simulink model "Total_90_NCKH"  (R2016a)
settings: Solver=FixedStepAuto  StartTime=0.0  StopTime=inf  RelTol=1e-3
libraries: arduinolib x12
settings Model: SimulationMode=external  ExtModeTrigDuration=2  Creator=Khuu Bach Thy  LastModifiedBy=ACER
settings OptimizationCC: OptimizeModelRefInitCode=on  LifeSpan=Inf  MaxStackSize=64
settings HardwareCC: ProdBitPerPointer=32  ProdLargestAtomicInteger=Long  ProdLargestAtomicFloat=Double  ProdWordSize=32  ProdHWDeviceType=ARM Compatible->ARM Cortex
settings RTWCC: SystemTargetFile=ert.tlc  HardwareBoard=Arduino Due  TemplateMakefile=ert_default_tmf  GenerateReport=on  Toolchain=Arduino ARM v1.6.1  BuildConfiguration=Faster Runs  IncludeHyperlinkInReport=on  LaunchReport=on  GenerateTraceInfo=on  GenerateTraceReport=on  GenerateTraceReportSl=on  GenerateTraceReportSf=on  GenerateTraceReportEml=on
settings CodeAppCC: ForceParamTrailComments=on  IgnoreCustomStorageClasses=off  OperatorAnnotations=on  SimulinkDataObjDesc=on  SFDataObjDesc=on  MATLABFcnDesc=on  MangleLength=10  InsertBlockDesc=on  MATLABSourceComments=on
settings ERTTargetCC: SupportContinuousTime=on  SupportVariableSizeSignals=on  ExtMode=on  ExtModeTransport=3  ExtModeMexFile=ext_serial_win32_comm_rtt  ExtModeMexArgs=0 10 115200

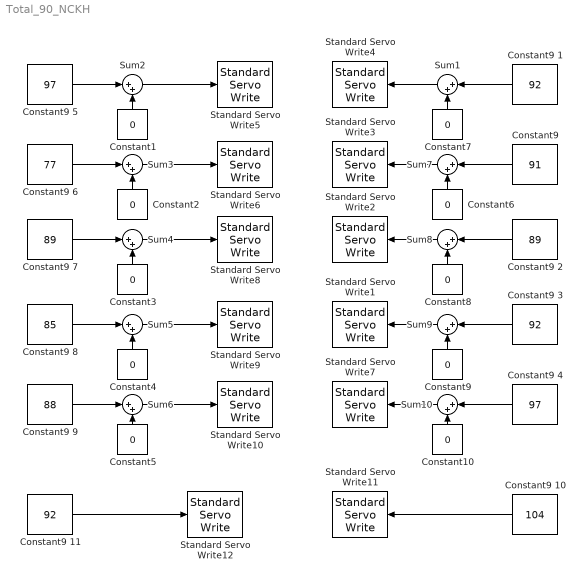
== system Total_90_NCKH ==
  Constant{1..10} (10 alike) : Constant  Value=0
  "Constant9 " : Constant  Value=91
  Constant9 1 : Constant  Value=92
  Constant9 10 : Constant  Value=104
  Constant9 11 : Constant  Value=92
  Constant9 2 : Constant  Value=89
  Constant9 3 : Constant  Value=92
  Constant9 4 : Constant  Value=97
  Constant9 5 : Constant  Value=97
  Constant9 6 : Constant  Value=77
  Constant9 7 : Constant  Value=89
  Constant9 8 : Constant  Value=85
  Constant9 9 : Constant  Value=88
  Standard Servo Write1 : arduinolib/Standard Servo Write  pinNumber=3  blockPlatform=arduino
  Standard Servo Write10 : arduinolib/Standard Servo Write  pinNumber=11  blockPlatform=arduino
  Standard Servo Write11 : arduinolib/Standard Servo Write  pinNumber=12  blockPlatform=arduino
  Standard Servo Write12 : arduinolib/Standard Servo Write  pinNumber=13  blockPlatform=arduino
  Standard Servo Write2 : arduinolib/Standard Servo Write  pinNumber=4  blockPlatform=arduino
  Standard Servo Write3 : arduinolib/Standard Servo Write  pinNumber=5  blockPlatform=arduino
  Standard Servo Write4 : arduinolib/Standard Servo Write  pinNumber=6  blockPlatform=arduino
  Standard Servo Write5 : arduinolib/Standard Servo Write  pinNumber=7  blockPlatform=arduino
  Standard Servo Write6 : arduinolib/Standard Servo Write  pinNumber=8  blockPlatform=arduino
  Standard Servo Write7 : arduinolib/Standard Servo Write  pinNumber=2  blockPlatform=arduino
  Standard Servo Write8 : arduinolib/Standard Servo Write  pinNumber=9  blockPlatform=arduino
  Standard Servo Write9 : arduinolib/Standard Servo Write  pinNumber=10  blockPlatform=arduino
  Sum{1..10} (10 alike) : Sum  Inputs=|++
  wires:
  Constant9 10/1 -> Standard Servo Write11/1
  Constant9 11/1 -> Standard Servo Write12/1
  Constant9 1/1 -> Sum1/1
  Sum1/1 -> Standard Servo Write4/1
  Sum2/1 -> Standard Servo Write5/1
  Constant9 5/1 -> Sum2/1
  Sum3/1 -> Standard Servo Write6/1
  Sum4/1 -> Standard Servo Write8/1
  Sum5/1 -> Standard Servo Write9/1
  Sum6/1 -> Standard Servo Write10/1
  Constant9 6/1 -> Sum3/1
  Constant9 7/1 -> Sum4/1
  Constant9 8/1 -> Sum5/1
  Constant9 9/1 -> Sum6/1
  Constant1/1 -> Sum2/2
  Constant2/1 -> Sum3/2
  Constant3/1 -> Sum4/2
  Constant5/1 -> Sum6/2
  Constant6/1 -> Sum7/2
  Constant7/1 -> Sum1/2
  "Constant9 "/1 -> Sum7/1
  Sum7/1 -> Standard Servo Write3/1
  Constant9 2/1 -> Sum8/1
  Sum8/1 -> Standard Servo Write2/1
  Constant8/1 -> Sum8/2
  Constant9 3/1 -> Sum9/1
  Sum9/1 -> Standard Servo Write1/1
  Constant9/1 -> Sum9/2
  Constant9 4/1 -> Sum10/1
  Sum10/1 -> Standard Servo Write7/1
  Constant10/1 -> Sum10/2
  Constant4/1 -> Sum5/2
